simulink model "sim7_2"  (R2019a)
settings: Solver=VariableStepAuto  StartTime=0.0  StopTime=10.0  RelTol=1e-3
values from neighbouring files (symbols this model uses):
  A = [0 1; -2 -3]    [matlab7_2.m]
  B = [0; 4]    [matlab7_2.m]
  C = [1 0]    [matlab7_2.m]
  Ca = [1 0;0 1]    [matlab7_2.m]
  D = 0    [matlab7_2.m]
  Da = [0; 0]    [matlab7_2.m]
  gamma = [0.0181; 0.3444]    [matlab7_2.m]
  h = 0.1    [matlab7_2.m]
  Lc = 1/(C*inv(eye(2)-phi_cl)*gamma)    [matlab7_2.m]
undefined symbols (not defined in the file or in its folder): L, phi
settings Model: Creator=User  LastModifiedBy=User

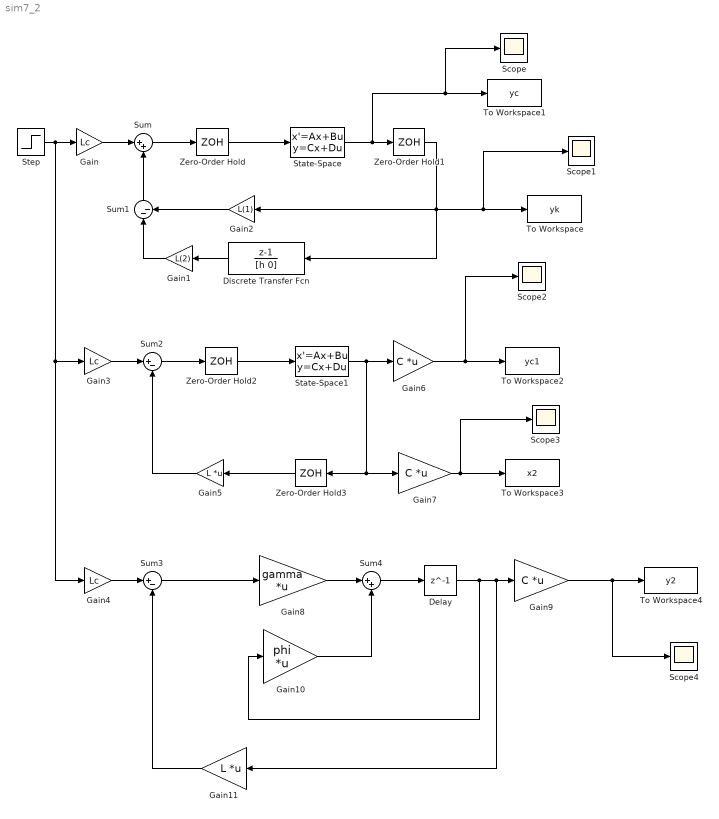
== system sim7_2 ==
  Delay : Delay  DelayLength=1
  Discrete Transfer Fcn : DiscreteTransferFcn  Numerator=[1 -1]  Denominator=[h 0]  SampleTime=h
  Gain : Gain  Gain=Lc
  Gain1 : Gain  Gain=L(2)
  Gain10 : Gain  Gain=phi  Multiplication=Matrix(K*u) (u vector)
  Gain11 : Gain  Gain=L  Multiplication=Matrix(K*u) (u vector)
  Gain2 : Gain  Gain=L(1)
  Gain3 : Gain  Gain=Lc
  Gain4 : Gain  Gain=Lc
  Gain5 : Gain  Gain=L  Multiplication=Matrix(K*u) (u vector)
  Gain6 : Gain  Gain=C  Multiplication=Matrix(K*u) (u vector)
  Gain7 : Gain  Gain=C  Multiplication=Matrix(K*u) (u vector)
  Gain8 : Gain  Gain=gamma  Multiplication=Matrix(K*u) (u vector)
  Gain9 : Gain  Gain=C  Multiplication=Matrix(K*u) (u vector)
  Scope{,1..4} (5 alike) : Scope
  State-Space : StateSpace  A=A  B=B  C=C  D=D  InitialCondition=0
  State-Space1 : StateSpace  A=A  B=B  C=Ca  D=Da  InitialCondition=0
  Step : Step  Time=0  SampleTime=0
  Sum : Sum  Inputs=|++
  Sum1 : Sum  Inputs=|--
  Sum2 : Sum  Inputs=|+-
  Sum3 : Sum  Inputs=|+-
  Sum4 : Sum  Inputs=|++
  To Workspace : ToWorkspace  VariableName=yk  SaveFormat=Structure With Time  SampleTime=-1
  To Workspace1 : ToWorkspace  VariableName=yc  SaveFormat=Structure With Time  SampleTime=-1
  To Workspace2 : ToWorkspace  VariableName=yc1  SaveFormat=Structure With Time  SampleTime=-1
  To Workspace3 : ToWorkspace  VariableName=x2  SaveFormat=Structure With Time  SampleTime=-1
  To Workspace4 : ToWorkspace  VariableName=y2  SaveFormat=Structure With Time  SampleTime=-1
  Zero-Order Hold{,1..3} (4 alike) : ZeroOrderHold  SampleTime=h
  wires:
  Step/1 -> Gain4/1, Gain3/1, Gain/1
  Gain/1 -> Sum/1
  Sum/1 -> Zero-Order Hold/1
  Zero-Order Hold/1 -> State-Space/1
  State-Space/1 -> Scope/1, To Workspace1/1, Zero-Order Hold1/1
  Zero-Order Hold1/1 -> Discrete Transfer Fcn/1, Scope1/1, To Workspace/1, Gain2/1
  Discrete Transfer Fcn/1 -> Gain1/1
  Gain1/1 -> Sum1/1
  Gain2/1 -> Sum1/2
  Sum1/1 -> Sum/2
  Sum2/1 -> Zero-Order Hold2/1
  Zero-Order Hold2/1 -> State-Space1/1
  Gain3/1 -> Sum2/1
  State-Space1/1 -> Zero-Order Hold3/1, Gain7/1, Gain6/1
  Gain6/1 -> Scope2/1, To Workspace2/1
  Gain7/1 -> Scope3/1, To Workspace3/1
  Zero-Order Hold3/1 -> Gain5/1
  Gain5/1 -> Sum2/2
  Gain4/1 -> Sum3/1
  Sum3/1 -> Gain8/1
  Gain8/1 -> Sum4/1
  Sum4/1 -> Delay/1
  Delay/1 -> Gain10/1, Gain11/1, Gain9/1
  Gain10/1 -> Sum4/2
  Gain11/1 -> Sum3/2
  Gain9/1 -> Scope4/1, To Workspace4/1
